simulink model "tank_ssr_safety_phase3"  (R2025b)
settings: Solver=ode45  StartTime=0.0  StopTime=3600  RelTol=1e-3
libraries: simulink x1, slpidlib x1
settings Model: Creator=maild  LastModifiedBy=maild

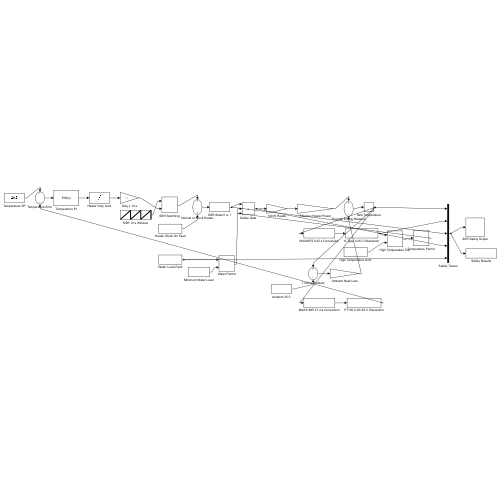
[thumbnail: Simulink's stored preview of the top-level diagram]
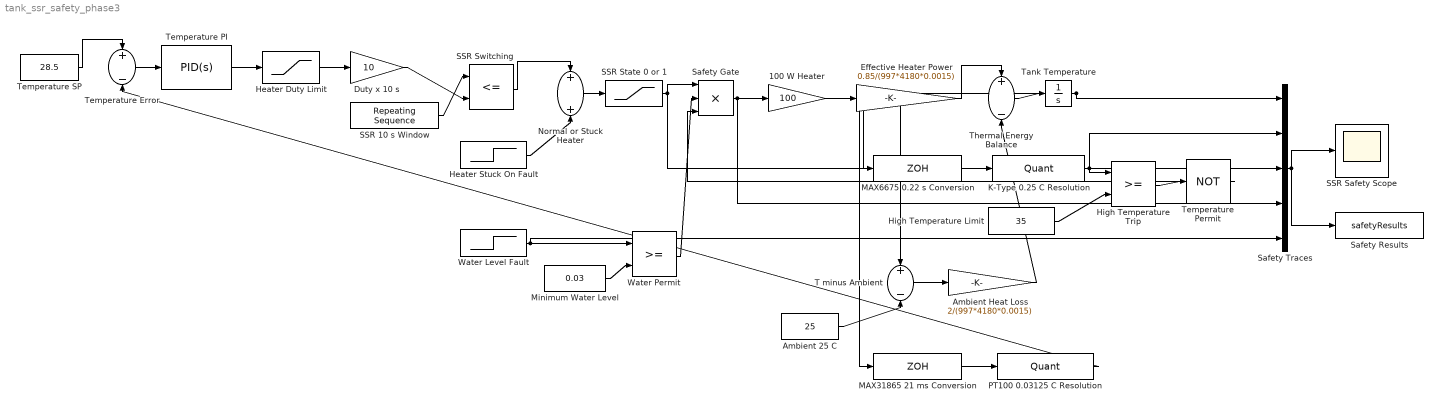
== system tank_ssr_safety_phase3 ==
  100 W Heater : Gain  Gain=100
  Ambient 25 C : Constant  Value=25
  Ambient Heat Loss : Gain  Gain=2/(997*4180*0.0015)
  Duty x 10 s : Gain  Gain=10
  Effective Heater Power : Gain  Gain=0.85/(997*4180*0.0015)
  Heater Duty Limit : Saturate  UpperLimit=0.10  LowerLimit=0
  Heater Stuck On Fault : Step  Time=1000  SampleTime=0
  High Temperature Limit : Constant  Value=35
  High Temperature Trip : RelationalOperator  OutDataTypeStr=boolean  RndMeth=Simplest  InputSameDT=off
  K-Type 0.25 C Resolution : Quantizer  QuantizationInterval=0.25
  MAX31865 21 ms Conversion : ZeroOrderHold  SampleTime=0.021
  MAX6675 0.22 s Conversion : ZeroOrderHold  SampleTime=0.22
  Minimum Water Level : Constant  Value=0.03
  Normal or Stuck Heater : Sum
  PT100 0.03125 C Resolution : Quantizer  QuantizationInterval=0.03125
  SSR 10 s Window : simulink/Sources/Repeating Sequence  rep_seq_t=[0 9.999 10]  rep_seq_y=[0 9.999 0]
  SSR Safety Scope : Scope
  SSR State 0 or 1 : Saturate  UpperLimit=1  LowerLimit=0
  SSR Switching : RelationalOperator  Operator=<=  OutDataTypeStr=boolean  RndMeth=Simplest  InputSameDT=off
  Safety Gate : Product  Inputs=3
  Safety Results : ToWorkspace  VariableName=safetyResults  SaveFormat=Structure With Time  SampleTime=-1
  Safety Traces : Mux  Inputs=5
  T minus Ambient : Sum  Inputs=+-
  Tank Temperature : Integrator  InitialCondition=25
  Temperature Error : Sum  Inputs=+-
  Temperature PI : slpidlib/PID Controller  Controller=PID  Form=Parallel  TimeDomain=Continuous-time  UseExternalTs=off  SampleTime=-1  IntegratorMethod=Forward Euler  FilterMethod=Forward Euler  ControllerParametersSource=internal  P=0.04  I=0.0008  UseKiTs=off  D=0  UseExternalDerivativeSource=off  N=100  UseFilter=on  TunerSelectOption=Transfer Function Based (PID Tuner App)  InitialConditionSource=internal  InitialConditionForIntegrator=0  InitialConditionForFilter=0  DifferentiatorICPrevScaledInput=0  ExternalReset=none  TrackingMode=off  Kt=1  LimitOutput=off  SatLimitsSource=internal  UpperSaturationLimit=inf  LowerSaturationLimit=-inf  LinearizeAsGain=on  AntiWindupMode=none  Kb=1  LimitIntegrator=off  UpperIntegratorSaturationLimit=inf  LowerIntegratorSaturationLimit=-inf  POutMin=[]  POutMax=[]  IOutMin=[]  IOutMax=[]  DOutMin=[]  DOutMax=[]  NOutMin=[]  NOutMax=[]  SumOutMin=[]  SumOutMax=[]  SaturationOutMin=[]  SaturationOutMax=[]  PParamMin=[]  PParamMax=[]  IParamMin=[]  IParamMax=[]  DParamMin=[]  DParamMax=[]  NParamMin=[]  NParamMax=[]  KbParamMin=[]  KbParamMax=[]  KtParamMin=[]  KtParamMax=[]  KbOutMin=[]  KbOutMax=[]  KtOutMin=[]  KtOutMax=[]  IntegratorOutMin=[]  IntegratorOutMax=[]  FilterOutMin=[]  FilterOutMax=[]  SumI1OutMin=[]  SumI1OutMax=[]  SumI2OutMin=[]  SumI2OutMax=[]  SumI3OutMin=[]  SumI3OutMax=[]  SumI4OutMin=[]  SumI4OutMax=[]  SumDOutMin=[]  SumDOutMax=[]  DifferentiatorOutMin=[]  DifferentiatorOutMax=[]  FilterDiffOutCoefMin=[]  FilterDiffOutCoefMax=[]  ReciprocalOutMin=[]  ReciprocalOutMax=[]  SumDenOutMin=[]  SumDenOutMax=[]  SumNumOutMin=[]  SumNumOutMax=[]  DivideOutMin=[]  DivideOutMax=[]  UdiffTsProdOutMin=[]  UdiffTsProdOutMax=[]  NTsProdOutMin=[]  NTsProdOutMax=[]  UintegralTsProdOutMin=[]  UintegralTsProdOutMax=[]  UngainTsProdOutMin=[]  UngainTsProdOutMax=[]  ClampingZeroOutDataTypeStr=Inherit: Inherit via back propagation  ClampingZeroOutMin=[]  ClampingZeroOutMax=[]  FilterDenConstantOutDataTypeStr=Inherit: Inherit via back propagation  FilterDenConstantOutMin=[]  FilterDenConstantOutMax=[]  PCopyOutDataTypeStr=Inherit: Inherit via back propagation  PCopyOutMin=[]  PCopyOutMax=[]  NCopyOutDataTypeStr=Inherit: Inherit via back propagation  NCopyOutMin=[]  NCopyOutMax=[]  IntegratorContinuousStateAttributes=''  IntegratorStateMustResolveToSignalObject=off  IntegratorRTWStateStorageClass=Auto  FilterContinuousStateAttributes=''  FilterStateMustResolveToSignalObject=off  FilterRTWStateStorageClass=Auto  ParallelPVariant=InternalParameters  IdealPVariant=Disabled  IVariant=InternalParameters  DVariant=InternalParameters  IntegratorVariant=Continuous  SatVariant=Disabled  AWVariant=Passthrough  PCopyVariant=Disabled  TRVariant=Disabled  FdbkBlocksVariant=Forward  IdealPFdbkVariant=Disabled  SatFdbkVariant=Disabled  DerivativeFilterVariant=ContFilter  NVariant=InternalParameters  NCopyVariant=Disabled  FilterICVariant=InternalICsFilter  IntegratorICVariant=InternalICs  ExternalResetVariant=Disabled  TRSumVariant=Passthrough  SumFdbkVariant=Disabled  SumVariant=Sum_PID  TsampFilterVariant=InternalTs  TsampNgainVariant=Passthrough  TsampIntegralVariant=Disabled_SignalSpec  ExternalSaturationOutDataTypeStr=Inherit: Same as second input  DerivativeSourceVariant=ErrorSignal  PreIntVariant=InternalPreInt
  Temperature Permit : Logic  Operator=NOT  AllPortsSameDT=off  OutDataTypeStr=boolean
  Temperature SP : Constant  Value=28.5
  Thermal Energy Balance : Sum  Inputs=+-
  Water Level Fault : Step  Time=2600  Before=0.08  After=0.01  SampleTime=0
  Water Permit : RelationalOperator  OutDataTypeStr=boolean  RndMeth=Simplest  InputSameDT=off
  wires:
  Temperature SP/1 -> Temperature Error/1
  Temperature Error/1 -> Temperature PI/1
  Temperature PI/1 -> Heater Duty Limit/1
  Heater Duty Limit/1 -> Duty x 10 s/1
  SSR 10 s Window/1 -> SSR Switching/1
  Duty x 10 s/1 -> SSR Switching/2
  SSR Switching/1 -> Normal or Stuck Heater/1
  Heater Stuck On Fault/1 -> Normal or Stuck Heater/2
  Normal or Stuck Heater/1 -> SSR State 0 or 1/1
  SSR State 0 or 1/1 -> Safety Gate/1, Safety Traces/3
  Water Level Fault/1 -> Water Permit/1, Safety Traces/5
  Minimum Water Level/1 -> Water Permit/2
  Water Permit/1 -> Safety Gate/2
  Safety Gate/1 -> 100 W Heater/1, Safety Traces/4
  100 W Heater/1 -> Effective Heater Power/1
  Effective Heater Power/1 -> Thermal Energy Balance/1
  Tank Temperature/1 -> T minus Ambient/1, MAX6675 0.22 s Conversion/1, MAX31865 21 ms Conversion/1, Safety Traces/1
  Ambient 25 C/1 -> T minus Ambient/2
  T minus Ambient/1 -> Ambient Heat Loss/1
  Ambient Heat Loss/1 -> Thermal Energy Balance/2
  Thermal Energy Balance/1 -> Tank Temperature/1
  MAX6675 0.22 s Conversion/1 -> K-Type 0.25 C Resolution/1
  K-Type 0.25 C Resolution/1 -> High Temperature Trip/1, Safety Traces/2
  High Temperature Limit/1 -> High Temperature Trip/2
  High Temperature Trip/1 -> Temperature Permit/1
  Temperature Permit/1 -> Safety Gate/3
  MAX31865 21 ms Conversion/1 -> PT100 0.03125 C Resolution/1
  PT100 0.03125 C Resolution/1 -> Temperature Error/2
  Safety Traces/1 -> SSR Safety Scope/1, Safety Results/1
